simulink library "forceslib"  (R2023a)
settings: Solver=VariableStepAuto  StartTime=0.0  StopTime=10.0  RelTol=1e-3
undefined symbols (not defined in the file or in its folder): forcesnlmpcblock_InitFcn, forcesnlmpcblockMultistage_InitFcn
(part 2 of 2)

== matlab function forceslib/FORCES ADAPTIVE MPC (Sparse QP)/MPC/Optimizer ==
  settings: updateMethod=DISCRETE  sampleTime=MPCstruct.Ts
  data: xkkm1 input double; lastmv input; xkkp1 output; moorx input; mv output; yref input; md input; extmv input; umin input; umax input; dumin input; dumax input; ymin input; ymax input; ywt input; uwt input; duwt input; ecrwt input; uref input; A input; B input; C input; D input; U input; Y input; X input; DX input; Pkk input; MPCstruct parameter; cost output; mvseq output; xseq output; yseq output; exitflag output; solvetime output; solverid output; xkk output; Pkk output
function [xkkp1,mv,cost,mvseq,xseq,yseq,exitflag,solvetime,solverid,xkk,Pkk] = fcn(xkkm1,lastmv,moorx,yref,md,extmv,umin,umax,dumin,dumax,ymin,ymax,ywt,uwt,duwt,ecrwt,uref,A,B,C,D,U,Y,X,DX,Pkk,MPCstruct)
    % Pre-allocate all the MEX block outputs for the simulation mode %#ok<*PREALL>
    [xkkp1,mv,cost,mvseq,xseq,yseq,exitflag,solvetime,solverid,xkk,Pkk] = mpcSparseSimulinkBlock(xkkm1,lastmv,moorx,yref,md,extmv,umin,umax,dumin,dumax,ymin,ymax,ywt,uwt,duwt,ecrwt,uref,A,B,C,D,U,Y,X,DX,Pkk,MPCstruct,MPCstruct.IsDummy,1);
end

== matlab function forceslib/FORCES LTV MPC (Sparse QP)/MPC/Optimizer ==
  settings: updateMethod=DISCRETE  sampleTime=MPCstruct.Ts
  data: xkkm1 input double; lastmv input; xkkp1 output; moorx input; mv output; yref input; md input; extmv input; umin input; umax input; dumin input; dumax input; ymin input; ymax input; ywt input; uwt input; duwt input; ecrwt input; uref input; A input; B input; C input; D input; U input; Y input; X input; DX input; Pkk input; MPCstruct parameter; cost output; mvseq output; xseq output; yseq output; exitflag output; solvetime output; solverid output; xkk output; Pkk output
function [xkkp1,mv,cost,mvseq,xseq,yseq,exitflag,solvetime,solverid,xkk,Pkk] = fcn(xkkm1,lastmv,moorx,yref,md,extmv,umin,umax,dumin,dumax,ymin,ymax,ywt,uwt,duwt,ecrwt,uref,A,B,C,D,U,Y,X,DX,Pkk,MPCstruct)
    % Pre-allocate all the MEX block outputs for the simulation mode %#ok<*PREALL>
    [xkkp1,mv,cost,mvseq,xseq,yseq,exitflag,solvetime,solverid,xkk,Pkk] = mpcSparseSimulinkBlock(xkkm1,lastmv,moorx,yref,md,extmv,umin,umax,dumin,dumax,ymin,ymax,ywt,uwt,duwt,ecrwt,uref,A,B,C,D,U,Y,X,DX,Pkk,MPCstruct,MPCstruct.IsDummy,2);
end

== matlab function forceslib/FORCES Nonlinear MPC/MPC/NLMPC ==
  settings: updateMethod=DISCRETE  sampleTime=blkData.Ts
  data: x input; mv output; ref input; lastMV input; md input; MVTarget input; MVMin input; MVMax input; OutputMin input; OutputMax input; MVRateMin input; MVRateMax input; StateMin input; StateMax input; OutputWeights input; MVWeights input; MVRateWeights input; ECRWeight input; cost output size=[1,1]; mvseq output size=[blkData.p+1 blkData.nmv]; xseq output size=[blkData.p+1 blkData.nx]; yseq output size=[blkData.p+1 blkData.ny]; nlpstatus output size=[1,1]; nlpsolvetime output; solverid output; Parameter input; MV0 input size=[blkData.p blkData.nmv]; X0 input size=[blkData.p blkData.nx]; blkData parameter; X0 output; MV0 output
function [mv, cost, mvseq, xseq, yseq, nlpstatus, nlpsolvetime, solverid, X0, MV0] = fcn(x, ref, lastMV, md, MVTarget, ...
    MVMin, MVMax, OutputMin, OutputMax, MVRateMin, MVRateMax, StateMin, StateMax, ...
    OutputWeights, MVWeights, MVRateWeights, ECRWeight, Parameter, MV0, X0, blkData)
    
    % Calls NLP solver for Nonlinear MPC block
    [mv, cost, mvseq, xseq, yseq, nlpstatus, nlpsolvetime, solverid, X0, MV0] = nlmpcSimulinkBlock(x, ref, lastMV, md, MVTarget, ...
        MVMin, MVMax, OutputMin, OutputMax, MVRateMin, MVRateMax, StateMin, StateMax, ...
        OutputWeights, MVWeights, MVRateWeights, ECRWeight, Parameter, MV0, X0, blkData);
end

== matlab function forceslib/FORCES Multistage Nonlinear MPC/MPC/Multistage NLMPC ==
  settings: updateMethod=DISCRETE  sampleTime=blkData.Ts
  data: x input; lastMV input; md input; mv output; stateparam input; stageparam input; MVMin input; MVMax input; MVRateMin input; MVRateMax input; StateMin input; StateMax input; xTerminal input; z0ext input; z0 input; cost output size=[1,1]; mvseq output size=[blkData.p+1 blkData.nmv]; xseq output size=[blkData.p+1 blkData.nx]; nlpstatus output size=[1,1]; nlpsolvetime output; solverid output; z0next output size=[blkData.nz 1]; blkData parameter
function [mv, cost, mvseq, xseq, nlpstatus, nlpsolvetime, solverid, z0next] = fcn(x, lastMV, md, stateparam, stageparam,...
    MVMin, MVMax, MVRateMin, MVRateMax, StateMin, StateMax, xTerminal, z0ext, z0, blkData)
    
    % Calls NLP solver for Nonlinear MPC block
    [mv, cost, mvseq, xseq, nlpstatus, nlpsolvetime, solverid, z0next] = nlmpcMultistageSimulinkBlock(x, lastMV, md, stateparam, stageparam,...
        MVMin, MVMax, MVRateMin, MVRateMax, StateMin, StateMax, xTerminal, z0ext, z0, blkData);
end

== matlab function forceslib/FORCES MPC (Sparse QP)/MPC/Optimizer ==
  settings: updateMethod=DISCRETE  sampleTime=MPCstruct.Ts
  data: xkkm1 input double; lastmv input; xkkp1 output; moorx input; mv output; yref input; md input; extmv input; umin input; umax input; dumin input; dumax input; ymin input; ymax input; ywt input; uwt input; duwt input; ecrwt input; uref input; Pkk input; MPCstruct parameter; cost output; mvseq output; xseq output; yseq output; exitflag output; solvetime output; solverid output; xkk output
function [xkkp1,mv,cost,mvseq,xseq,yseq,exitflag,solvetime,solverid,xkk] = fcn(xkkm1,lastmv,moorx,yref,md,extmv,umin,umax,dumin,dumax,ymin,ymax,ywt,uwt,duwt,ecrwt,uref,Pkk,MPCstruct)
    % Pre-allocate all the MEX block outputs for the simulation mode %#ok<*PREALL>
    [xkkp1,mv,cost,mvseq,xseq,yseq,exitflag,solvetime,solverid,xkk,~] = mpcSparseSimulinkBlock(xkkm1,lastmv,moorx,yref,md,extmv,umin,umax,dumin,dumax,ymin,ymax,ywt,uwt,duwt,ecrwt,uref,0,0,0,0,0,0,0,0,Pkk,MPCstruct,MPCstruct.IsDummy,0);
end
